simulink model "QuarterCar_1DOF"  (R2025b)
settings: Solver=VariableStepAuto  StartTime=0.0  StopTime=10.0  RelTol=1e-3
settings Model: Creator=Aditya  LastModifiedBy=Aditya

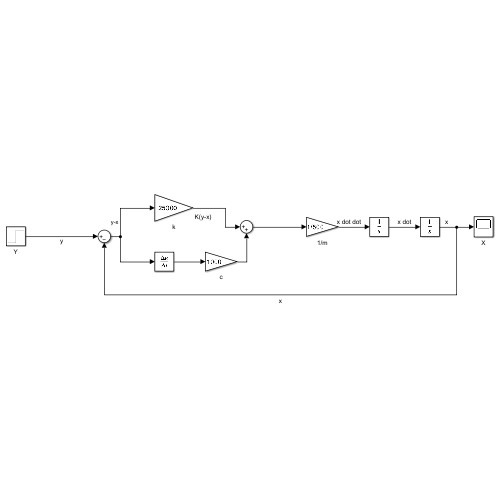
[thumbnail: Simulink's stored preview of the top-level diagram]
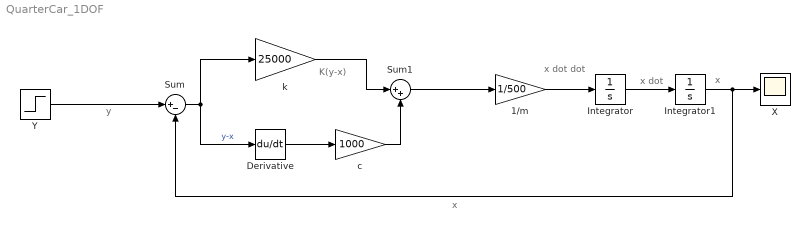
== system QuarterCar_1DOF ==
  note: x
  note: x
  note: x dot
  note: x dot dot
  note: K(y-x)
  note: y
  1/m : Gain  Gain=1/500
  Derivative : Derivative
  Integrator : Integrator
  Integrator1 : Integrator
  Sum : Sum  Inputs=|+-
  Sum1 : Sum  Inputs=|++
  X : Scope
      settings: ActiveDisplayYMinimum=-0.10180721143980817  ActiveDisplayYMaximum=0.91626490295827379
  Y : Step  After=0.5  SampleTime=0
  c : Gain  Gain=1000
  k : Gain  Gain=25000
  wires:
  Y/1 -> Sum/1
  Integrator1/1 -> Sum/2, X/1
  Sum/1 -> Derivative/1, k/1  "y-x"
  k/1 -> Sum1/1
  Derivative/1 -> c/1
  c/1 -> Sum1/2
  Sum1/1 -> 1/m/1
  1/m/1 -> Integrator/1
  Integrator/1 -> Integrator1/1
